simulink model "ActiveSuspensionController"  (R2022a)
settings: Solver=ode1  StartTime=0.0  StopTime=10.0  FixedStep=0.001  RelTol=1e-3
values from neighbouring files (symbols this model uses):
  A_observer = A-G*C    [ActiveSuspensionScript.m]
  B_observer = [G B]    [ActiveSuspensionScript.m]
  K = lqr(A,B,Q,R,N)    [ActiveSuspensionScript.m]
settings Model: Creator=burl  LastModifiedBy=prajw
settings SolverCC: AlgebraicLoopSolver=TrustRegion
settings DataIOCC: ReturnWorkspaceOutputs=off
settings DebuggingCC: UnconnectedInputMsg=warning  UnconnectedOutputMsg=warning  UnconnectedLineMsg=warning  SFMachineParentedDataDiag=warning  ArithmeticOperatorsInVariantConditions=warning
settings SFSimCC: SimUseLocalCustomCode=off  CustomCodeUndefinedFunction=UseInterfaceOnly
settings RTWCC: RTWUseLocalCustomCode=off

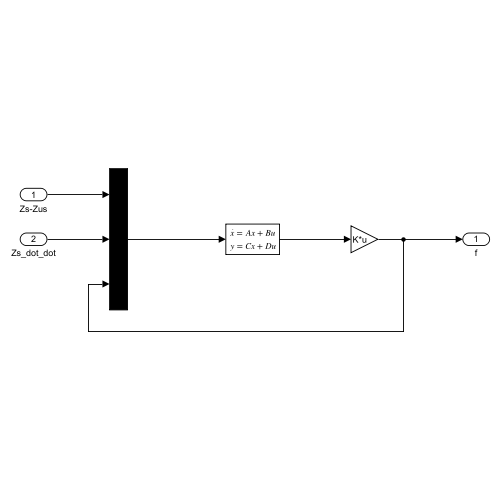
[thumbnail: Simulink's stored preview of the top-level diagram]
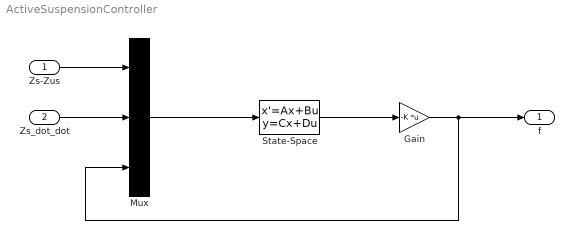
== system ActiveSuspensionController ==
  Zs-Zus : Inport
  Zs_dot_dot : Inport  Port=2
  Gain : Gain  Gain=-K  Multiplication=Matrix(K*u)
  Mux : Mux  Inputs=3
  State-Space : StateSpace  A=A_observer  B=B_observer  C=[1 0 0 0; 0 1 0 0; 0 0 1 0; 0 0 0 1]  D="[0 0 0 ;  0 0 0;  0 0 0; 0 0 0]"  InitialCondition=0
  f : Outport  VectorParamsAs1DForOutWhenUnconnected=off
  wires:
  Zs-Zus/1 -> Mux/1
  Zs_dot_dot/1 -> Mux/2
  Mux/1 -> State-Space/1
  State-Space/1 -> Gain/1
  Gain/1 -> Mux/3, f/1
